simulink library "periodicCtrlExpStateMachine"  (R2020a)
settings: Solver=VariableStepAuto  StartTime=0.0  StopTime=10.0  RelTol=1e-3
undefined symbols (not defined in the file or in its folder): fltCtrl, initializeBussesFromBlock
libraries: dspsigops x3, simulink x2, $bdroot x1
settings Model: Creator=jcreed2  LastModifiedBy=jcreed2

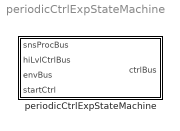
== system periodicCtrlExpStateMachine ==
  periodicCtrlExpStateMachine : Subsystem  LoadFcn=initializeBussesFromBlock(gcb)  InitFcn=initializeBussesFromBlock(gcb)  mask{fltCtrl=fltCtrl}
      mask prompts: fltCtrl "Controller Model"

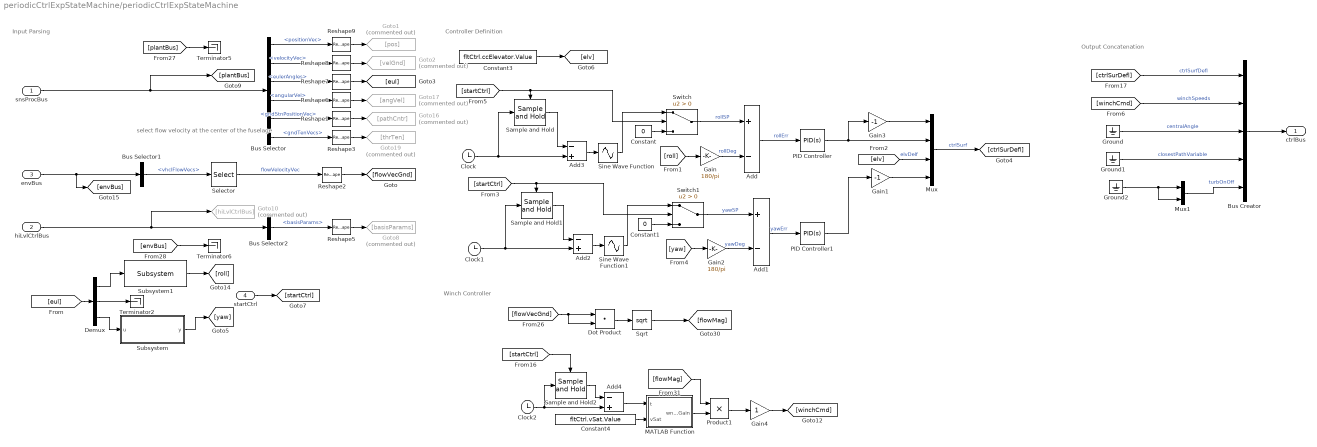
== system periodicCtrlExpStateMachine/periodicCtrlExpStateMachine ==
  note: Winch Controller
  note: Controller Definition
  note: select flow velocity at the center of the fuselage
  note: Input Parsing
  note: Output Concatenation
  snsProcBus : Inport  OutDataTypeStr=Bus: sensorsProcessingBus
  hiLvlCtrlBus : Inport  Port=2  OutDataTypeStr=Bus: hiLvlCtrlBus
  envBus : Inport  Port=3  OutDataTypeStr=Bus: envBus
  startCtrl : Inport  Port=4
  Add : Sum  Inputs=+-
  Add1 : Sum  Inputs=+-
  Add2 : Sum  Inputs=-+
  Add3 : Sum  Inputs=-+
  Add4 : Sum  Inputs=-+
  Bus Creator : BusCreator  Inputs=5  OutDataTypeStr=Bus: fltCtrlBus
      settings: InheritFromInputs=off
  Bus Selector : BusSelector  OutputSignals=positionVec,velocityVec,eulerAngles,angularVel,gndStnPositionVec,gndTenVecs
  Bus Selector1 : BusSelector  OutputSignals=vhclFlowVecs
  Bus Selector2 : BusSelector  OutputSignals=basisParams
  Clock : Clock
  Clock1 : Clock
  Clock2 : Clock
  Constant : Constant  Value=0
  Constant1 : Constant  Value=0
  Constant3 : Constant  Value=fltCtrl.ccElevator.Value
  Constant4 : Constant  Value=fltCtrl.vSat.Value
  Demux : Demux  Outputs=3
  Dot Product : DotProduct  InputSameDT=on  OutDataTypeStr=Inherit: Inherit via internal rule
  Gain : Gain  Gain=180/pi
  Gain1 : Gain  Gain=-1
  Gain2 : Gain  Gain=180/pi
  Gain3 : Gain  Gain=-1
  Gain4 : Gain
  Goto1 : Goto  Commented=on  GotoTag=pos
  Goto10 : Goto  Commented=on  GotoTag=hiLvlCtrlBus
  Goto16 : Goto  Commented=on  GotoTag=pathCntr
  Goto17 : Goto  Commented=on  GotoTag=angVel
  Goto19 : Goto  Commented=on  GotoTag=thrTen
  Goto2 : Goto  Commented=on  GotoTag=velGnd
  Goto8 : Goto  Commented=on  GotoTag=basisParams
  Ground : Ground
  Ground1 : Ground
  Ground2 : Ground
  MATLAB Function : MATLAB Function  TreatAsAtomicUnit=on
  Mux : Mux
  Mux1 : Mux  Inputs=2
  PID Controller : simulink/Continuous/PID Controller  Controller=PID  Form=Parallel  TimeDomain=Continuous-time  UseExternalTs=off  SampleTime=-1  IntegratorMethod=Forward Euler  FilterMethod=Forward Euler  ControllerParametersSource=internal  P=fltCtrl.rollCtrl.kp.Value  I=0  D=fltCtrl.rollCtrl.kd.Value  UseFilter=on  N=fltCtrl.rollCtrl.tau.Value  TunerSelectOption=Transfer Function Based (PID Tuner App)  InitialConditionSource=internal  InitialConditionForIntegrator=0  InitialConditionForFilter=0  DifferentiatorICPrevScaledInput=0  ExternalReset=none  TrackingMode=off  Kt=1  LimitOutput=off  UpperSaturationLimit=inf  LowerSaturationLimit=-inf  LinearizeAsGain=on  AntiWindupMode=none  Kb=1  POutMin=[]  POutMax=[]  IOutMin=[]  IOutMax=[]  DOutMin=[]  DOutMax=[]  NOutMin=[]  NOutMax=[]  SumOutMin=[]  SumOutMax=[]  SaturationOutMin=[]  SaturationOutMax=[]  PParamMin=[]  PParamMax=[]  IParamMin=[]  IParamMax=[]  DParamMin=[]  DParamMax=[]  NParamMin=[]  NParamMax=[]  KbParamMin=[]  KbParamMax=[]  KtParamMin=[]  KtParamMax=[]  KbOutMin=[]  KbOutMax=[]  KtOutMin=[]  KtOutMax=[]  IntegratorOutMin=[]  IntegratorOutMax=[]  FilterOutMin=[]  FilterOutMax=[]  SumI1OutMin=[]  SumI1OutMax=[]  SumI2OutMin=[]  SumI2OutMax=[]  SumI3OutMin=[]  SumI3OutMax=[]  SumI4OutMin=[]  SumI4OutMax=[]  SumDOutMin=[]  SumDOutMax=[]  DifferentiatorOutMin=[]  DifferentiatorOutMax=[]  FilterDiffOutCoefMin=[]  FilterDiffOutCoefMax=[]  ReciprocalOutMin=[]  ReciprocalOutMax=[]  SumDenOutMin=[]  SumDenOutMax=[]  SumNumOutMin=[]  SumNumOutMax=[]  DivideOutMin=[]  DivideOutMax=[]  UdiffTsProdOutMin=[]  UdiffTsProdOutMax=[]  NTsProdOutMin=[]  NTsProdOutMax=[]  UintegralTsProdOutMin=[]  UintegralTsProdOutMax=[]  UngainTsProdOutMin=[]  UngainTsProdOutMax=[]  IntegratorContinuousStateAttributes=''  IntegratorStateMustResolveToSignalObject=off  IntegratorRTWStateStorageClass=Auto  FilterContinuousStateAttributes=''  FilterStateMustResolveToSignalObject=off  FilterRTWStateStorageClass=Auto  ParallelPVariant=InternalParameters  IdealPVariant=Disabled  IVariant=InternalParameters  DVariant=InternalParameters  IntegratorVariant=Continuous  SatVariant=Disabled  AWVariant=Passthrough  PCopyVariant=Disabled  TRVariant=Disabled  FdbkBlocksVariant=Forward  IdealPFdbkVariant=Disabled  SatFdbkVariant=Disabled  DerivativeFilterVariant=ContFilter  NVariant=InternalParameters  NCopyVariant=Disabled  FilterICVariant=InternalICsFilter  IntegratorICVariant=InternalICs  ExternalResetVariant=Disabled  TRSumVariant=Passthrough  SumFdbkVariant=Disabled  SumVariant=Sum_PID  TsampFilterVariant=InternalTs  TsampNgainVariant=Passthrough  TsampIntegralVariant=Passthrough
  PID Controller1 : simulink/Continuous/PID Controller  Controller=PID  Form=Parallel  TimeDomain=Continuous-time  UseExternalTs=off  SampleTime=-1  IntegratorMethod=Forward Euler  FilterMethod=Forward Euler  ControllerParametersSource=internal  P=fltCtrl.yawCtrl.kp.Value  I=0  D=fltCtrl.yawCtrl.kd.Value  UseFilter=on  N=fltCtrl.yawCtrl.tau.Value  TunerSelectOption=Transfer Function Based (PID Tuner App)  InitialConditionSource=internal  InitialConditionForIntegrator=0  InitialConditionForFilter=0  DifferentiatorICPrevScaledInput=0  ExternalReset=none  TrackingMode=off  Kt=1  LimitOutput=off  UpperSaturationLimit=inf  LowerSaturationLimit=-inf  LinearizeAsGain=on  AntiWindupMode=none  Kb=1  POutMin=[]  POutMax=[]  IOutMin=[]  IOutMax=[]  DOutMin=[]  DOutMax=[]  NOutMin=[]  NOutMax=[]  SumOutMin=[]  SumOutMax=[]  SaturationOutMin=[]  SaturationOutMax=[]  PParamMin=[]  PParamMax=[]  IParamMin=[]  IParamMax=[]  DParamMin=[]  DParamMax=[]  NParamMin=[]  NParamMax=[]  KbParamMin=[]  KbParamMax=[]  KtParamMin=[]  KtParamMax=[]  KbOutMin=[]  KbOutMax=[]  KtOutMin=[]  KtOutMax=[]  IntegratorOutMin=[]  IntegratorOutMax=[]  FilterOutMin=[]  FilterOutMax=[]  SumI1OutMin=[]  SumI1OutMax=[]  SumI2OutMin=[]  SumI2OutMax=[]  SumI3OutMin=[]  SumI3OutMax=[]  SumI4OutMin=[]  SumI4OutMax=[]  SumDOutMin=[]  SumDOutMax=[]  DifferentiatorOutMin=[]  DifferentiatorOutMax=[]  FilterDiffOutCoefMin=[]  FilterDiffOutCoefMax=[]  ReciprocalOutMin=[]  ReciprocalOutMax=[]  SumDenOutMin=[]  SumDenOutMax=[]  SumNumOutMin=[]  SumNumOutMax=[]  DivideOutMin=[]  DivideOutMax=[]  UdiffTsProdOutMin=[]  UdiffTsProdOutMax=[]  NTsProdOutMin=[]  NTsProdOutMax=[]  UintegralTsProdOutMin=[]  UintegralTsProdOutMax=[]  UngainTsProdOutMin=[]  UngainTsProdOutMax=[]  IntegratorContinuousStateAttributes=''  IntegratorStateMustResolveToSignalObject=off  IntegratorRTWStateStorageClass=Auto  FilterContinuousStateAttributes=''  FilterStateMustResolveToSignalObject=off  FilterRTWStateStorageClass=Auto  ParallelPVariant=InternalParameters  IdealPVariant=Disabled  IVariant=InternalParameters  DVariant=InternalParameters  IntegratorVariant=Continuous  SatVariant=Disabled  AWVariant=Passthrough  PCopyVariant=Disabled  TRVariant=Disabled  FdbkBlocksVariant=Forward  IdealPFdbkVariant=Disabled  SatFdbkVariant=Disabled  DerivativeFilterVariant=ContFilter  NVariant=InternalParameters  NCopyVariant=Disabled  FilterICVariant=InternalICsFilter  IntegratorICVariant=InternalICs  ExternalResetVariant=Disabled  TRSumVariant=Passthrough  SumFdbkVariant=Disabled  SumVariant=Sum_PID  TsampFilterVariant=InternalTs  TsampNgainVariant=Passthrough  TsampIntegralVariant=Passthrough
  Product1 : Product
  Reshape{1..3,5..9} (8 alike) : Reshape  OutputDimensionality=Column vector (2-D)
  Sample and Hold : dspsigops/Sample and Hold  trig=Rising edge  initCond=0  latchinput=off
  Sample and Hold1 : dspsigops/Sample and Hold  trig=Rising edge  initCond=0  latchinput=off
  Sample and Hold2 : dspsigops/Sample and Hold  trig=Rising edge  initCond=0  latchinput=off
  Selector : Selector  NumberOfDimensions=2  InputPortWidth=3  IndexOptions=Select all,Index vector (dialog)  Indices=[1 3],5  OutputSizes=1,1
  Sine Wave Function : Sin  TimeSource=Use external signal  Amplitude=fltCtrl.rollAmp.Value  Frequency=fltCtrl.frequency.Value  Phase=fltCtrl.rollPhase.Value  SampleTime=0
  Sine Wave Function1 : Sin  TimeSource=Use external signal  Amplitude=fltCtrl.yawAmp.Value  Frequency=fltCtrl.frequency.Value  Phase=fltCtrl.yawPhase.Value  SampleTime=0
  Sqrt : Sqrt  SaturateOnIntegerOverflow=on
  Subsystem : Subsystem
  Subsystem1 : $bdroot/periodicCtrlExpStateMachine/Subsystem  SystemSampleTime=-1  Latency=0  AutoFrameSizeCalculation=off
  Switch : Switch  Criteria=u2 > Threshold
  Switch1 : Switch  Criteria=u2 > Threshold
  Terminator2 : Terminator
  Terminator5 : Terminator
  Terminator6 : Terminator
  ctrlBus : Outport  OutDataTypeStr=Bus: fltCtrlBus  VectorParamsAs1DForOutWhenUnconnected=off
  wires:
  Reshape1/1 -> Goto16/1
  Reshape9/1 -> Goto1/1
  Bus Selector/5 -> Reshape1/1  "<gndStnPositionVec>"
  Bus Selector/3 -> Reshape7/1  "<eulerAngles>"
  Demux/2 -> Terminator2/1
  [envBus] -> Terminator6/1
  Reshape3/1 -> Goto19/1
  Reshape5/1 -> Goto8/1
  envBus/1 -> [envBus], Bus Selector1/1
  Bus Creator/1 -> ctrlBus/1
  Bus Selector/1 -> Reshape9/1  "<positionVec>"
  [winchCmd] -> Bus Creator/2  "winchSpeeds"
  Bus Selector/4 -> Reshape6/1  "<angularVel>"
  Reshape6/1 -> Goto17/1
  Bus Selector2/1 -> Reshape5/1  "<basisParams>"
  Bus Selector/2 -> Reshape8/1  "<velocityVec>"
  Reshape2/1 -> [flowVecGnd]
  [ctrlSurDefl] -> Bus Creator/1  "ctrlSurfDefl"
  [elv] -> Mux/3  "elvDelf"
  [plantBus] -> Terminator5/1
  Reshape7/1 -> [eul]
  Selector/1 -> Reshape2/1  "flowVelocityVec"
  [eul] -> Demux/1
  Bus Selector/6 -> Reshape3/1  "<gndTenVecs>"
  Demux/1 -> Subsystem1/1
  Demux/3 -> Subsystem/1(u)
  Reshape8/1 -> Goto2/1
  Bus Selector1/1 -> Selector/1  "<vhclFlowVecs>"
  [roll] -> Gain/1
  Add/1 -> PID Controller/1  "rollErr"
  Gain/1 -> Add/2  "rollDeg"
  Clock/1 -> Add3/2, Sample and Hold/1
  Mux/1 -> [ctrlSurDefl]  "ctrlSurf"
  Constant3/1 -> [elv]
  Sample and Hold/1 -> Add3/1
  Add3/1 -> Sine Wave Function/1
  Sine Wave Function/1 -> Switch/1
  [startCtrl] -> Switch/2, Sample and Hold/Trigger
  Constant/1 -> Switch/3
  Switch/1 -> Add/1  "rollSP"
  Ground/1 -> Bus Creator/3  "centralAngle"
  Ground1/1 -> Bus Creator/4  "closestPathVariable"
  Ground2/1 -> Mux1/2, Mux1/1
  Mux1/1 -> Bus Creator/5  "turbOnOff"
  [startCtrl] -> Sample and Hold1/Trigger, Switch1/2
  Constant1/1 -> Switch1/3
  Switch1/1 -> Add1/1  "yawSP"
  Add2/1 -> Sine Wave Function1/1
  Gain2/1 -> Add1/2  "yawDeg"
  [yaw] -> Gain2/1
  Sample and Hold1/1 -> Add2/1
  Clock1/1 -> Sample and Hold1/1, Add2/2
  Add1/1 -> PID Controller1/1  "yawErr"
  snsProcBus/1 -> Bus Selector/1, [plantBus]
  hiLvlCtrlBus/1 -> Goto10/1, Bus Selector2/1
  PID Controller1/1 -> Gain1/1
  Sine Wave Function1/1 -> Switch1/1
  PID Controller/1 -> Mux/2, Gain3/1
  Gain1/1 -> Mux/4
  Gain3/1 -> Mux/1
  startCtrl/1 -> [startCtrl]
  Clock2/1 -> Add4/2, Sample and Hold2/1
  MATLAB Function/1(wnchGain) -> Product1/2
  [flowMag] -> Product1/1
  Product1/1 -> Gain4/1
  Constant4/1 -> MATLAB Function/2(vSat)
  [startCtrl] -> Sample and Hold2/Trigger
  Add4/1 -> MATLAB Function/1(t)
  Sample and Hold2/1 -> Add4/1
  Sqrt/1 -> [flowMag]
  Dot Product/1 -> Sqrt/1
  [flowVecGnd] -> Dot Product/2, Dot Product/1
  Subsystem/1(y) -> [yaw]
  Subsystem1/1 -> [roll]
  Gain4/1 -> [winchCmd]

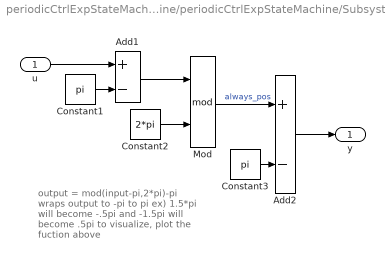
== system periodicCtrlExpStateMachine/periodicCtrlExpStateMachine/Subsystem ==
  note: output = mod(input-pi,2*pi)-pi
      | wraps output to -pi to pi
      |
      | ex) 1.5*pi will become -.5pi
      | 	and -1.5pi will become .5pi
      |
      | to visualize, plot the fuction above
  u : Inport
  Add1 : Sum  Inputs=+-
  Add2 : Sum  Inputs=+-
  Constant1 : Constant  Value=pi
  Constant2 : Constant  Value=2*pi
  Constant3 : Constant  Value=pi
  Mod : Math  Operator=mod  SignedPower=on  SaturateOnIntegerOverflow=on
  y : Outport  VectorParamsAs1DForOutWhenUnconnected=off
  wires:
  Constant3/1 -> Add2/2
  Add2/1 -> y/1
  u/1 -> Add1/1
  Constant1/1 -> Add1/2
  Constant2/1 -> Mod/2
  Mod/1 -> Add2/1  "always_pos"
  Add1/1 -> Mod/1

== matlab function periodicCtrlExpStateMachine/MATLAB Function ==
  data: t input; wnchGain output; vSat input
function wnchGain   = fcn(t,vSat)
wnchGain = 0;
if t< 15 || t>150
    wnchGain = 0;
else
    wnchGain = .001*(t-15)^2;
end

if wnchGain >= vSat
    wnchGain = vSat;
end
